simulink model "reducedorderobserver"  (R2023a)
settings: Solver=VariableStepAuto  StartTime=0.0  StopTime=10.0  RelTol=1e-3
values from neighbouring files (symbols this model uses):
  A = [0 0 1 0 0 ... (first row only)    [obsv_ctrb.m]    (also in reduced_order.m = [0 0 1 0)
  A_aa = A(1:2, 1:2)    [observer_design.m]
  A_ab = A(1:2, 3:4)    [observer_design.m]
  A_ba = A(3:4, 1:2)    [observer_design.m]
  A_bb = A(3:4, 3:4)    [observer_design.m]
  B = [0; 0; 0; 0; 1/L_a]    [obsv_ctrb.m]    (also in reduced_order.m = [0; 0; K_m/(J_m * R); 0])
  B_a = B(1:2, :)    [observer_design.m]
  B_b = B(3:4, :)    [observer_design.m]
  C = [0 1 0 0 0]    [obsv_ctrb.m]    (also in reduced_order.m = [0 1 0 0]; testobsv.m = [1 0 0 0 0])
  C_o = [1 0 0 0 ... (first row only)    [observer_design.m]
  K_cont_int = K_cont(1,1)    [polesplacement.m]
  K_cont_x = K_cont(1, 2:5)    [polesplacement.m]
  K_disc_int = K_disc(1,1)    [polesplacement.m]
  K_disc_x = K_disc(1, 2:5)    [polesplacement.m]
  L_r = place(A_bb', A_ab', [closest_pole, closest_pole+1])'    [observer_design.m]
  sys_disc = c2d(sys, min_sampling_time, "zoh")    [polesplacement.m]
  x1_bar = deg2rad(31.78)    [reduced_order.m]
  x2_bar = deg2rad(30)    [reduced_order.m]
undefined symbols (not defined in the file or in its folder): g, I_noload, init, K_m, l, m, min_sampling_time, R
libraries: simulink x2
settings Model: Creator=yunzh  LastModifiedBy=yunzh

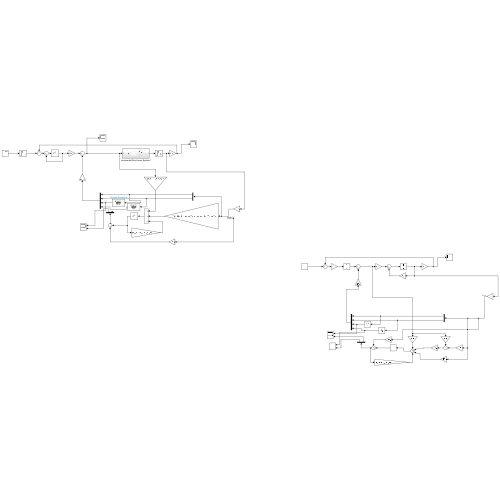
[thumbnail: Simulink's stored preview of the top-level diagram]
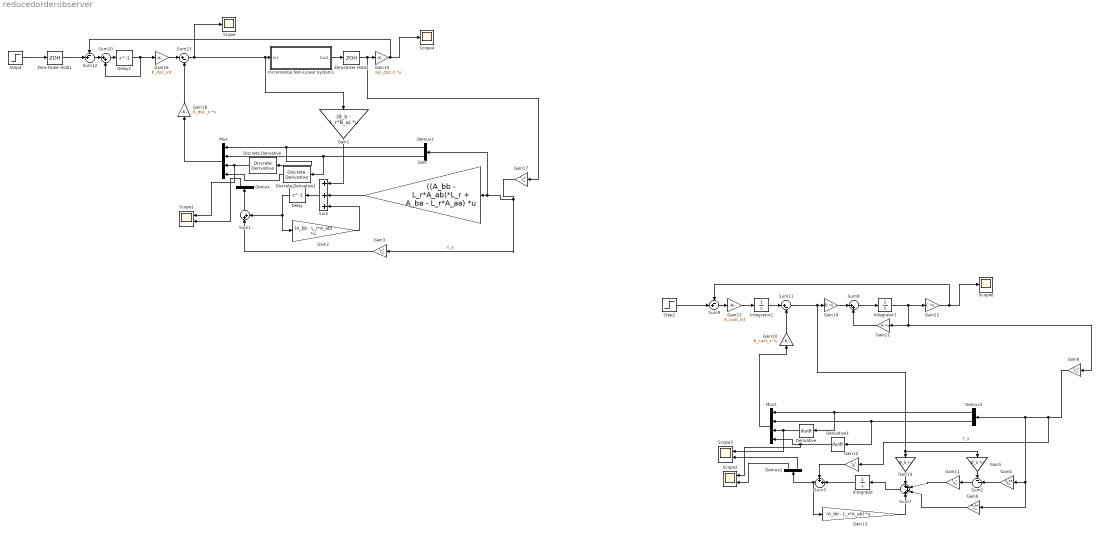
== system reducedorderobserver ==
  Delay : Delay  DelayLength=1
  Delay2 : Delay  DelayLength=1  SampleTime=min_sampling_time
  Demux{,1..3} (4 alike) : Demux  Outputs=2
  Derivative : Derivative
  Derivative1 : Derivative
  Discrete Derivative : simulink/Discrete/Discrete Derivative  gainval=1.0  ICPrevScaledInput=0.0  OutMin=[]  OutMax=[]  OutDataType=fixdt(1, 16)  OutScaling=2^-10  DoSatur=off
  Discrete Derivative1 : simulink/Discrete/Discrete Derivative  gainval=1.0  ICPrevScaledInput=0.0  OutMin=[]  OutMax=[]  OutDataType=fixdt(1, 16)  OutScaling=2^-10  DoSatur=off
  Gain : Gain  Gain=((A_bb - L_r*A_ab)*L_r + A_ba - L_r*A_aa)  Multiplication=Matrix(K*u)
  Gain1 : Gain  Gain=(B_b - L_r*B_a)  Multiplication=Matrix(K*u)
  Gain10 : Gain  Gain=B_b  Multiplication=Matrix(K*u)
  Gain11 : Gain  Gain=L_r  Multiplication=Matrix(K*u)
  Gain12 : Gain  Gain=L_r  Multiplication=Matrix(K*u)
  Gain13 : Gain  Gain=(A_bb - L_r*A_ab)  Multiplication=Matrix(K*u)
  Gain15 : Gain  Gain=sys_disc.C  Multiplication=Matrix(K*u)
  Gain16 : Gain  Gain=K_disc_int
  Gain17 : Gain  Gain=C_o  Multiplication=Matrix(K*u)
  Gain18 : Gain  Gain=K_disc_x  Multiplication=Matrix(K*u)
  Gain19 : Gain  Gain=B  Multiplication=Matrix(K*u)
  Gain2 : Gain  Gain=(A_bb - L_r*A_ab)  Multiplication=Matrix(K*u)
  Gain20 : Gain  Gain=K_cont_x  Multiplication=Matrix(K*u)
  Gain21 : Gain  Gain=A  Multiplication=Matrix(K*u)
  Gain22 : Gain  Gain=C  Multiplication=Matrix(K*u)
  Gain23 : Gain  Gain=K_cont_int
  Gain3 : Gain  Gain=L_r  Multiplication=Matrix(K*u)
  Gain4 : Gain  Gain=A_aa  Multiplication=Matrix(K*u)
  Gain5 : Gain  Gain=B_a  Multiplication=Matrix(K*u)
  Gain6 : Gain  Gain=A_ba  Multiplication=Matrix(K*u)
  Gain8 : Gain  Gain=C_o  Multiplication=Matrix(K*u)
  Incremental Non-Linear System1 : Subsystem
  Integrator : Integrator
  Integrator1 : Integrator
  Integrator2 : Integrator
  Mux : Mux
  Mux1 : Mux
  Scope : Scope
  Scope1 : Scope  NumInputPorts=2
  Scope2 : Scope  NumInputPorts=2
  Scope3 : Scope  NumInputPorts=2
  Scope4 : Scope
  Scope6 : Scope
  Step2 : Step  Time=0  After=0.5  SampleTime=0
  Step4 : Step  Time=0  After=deg2rad(15)  SampleTime=min_sampling_time
  Sum : Sum  Inputs=+++
  Sum1 : Sum  Inputs=|++
  Sum10 : Sum  Inputs=|++
  Sum11 : Sum  Inputs=|+-
  Sum12 : Sum  Inputs=-+|
  Sum13 : Sum  Inputs=|+-
  Sum2 : Sum  Inputs=--|
  Sum3 : Sum  Inputs=++|
  Sum7 : Sum  Inputs=++++
  Sum8 : Sum  Inputs=|++
  Sum9 : Sum  Inputs=-+|
  Zero-Order Hold1 : ZeroOrderHold  SampleTime=min_sampling_time
  Zero-Order Hold2 : ZeroOrderHold  SampleTime=-1
  wires:
  Gain18/1 -> Sum13/2
  Zero-Order Hold2/1 -> Gain17/1, Gain15/1
  Gain17/1 -> Gain3/1, Demux1/1, Gain/1  "X_a"
  Incremental Non-Linear System1/1(Out1) -> Zero-Order Hold2/1
  Sum13/1 -> Scope/1, Gain1/1, Incremental Non-Linear System1/1(In1)
  Zero-Order Hold1/1 -> Sum12/2
  Step4/1 -> Zero-Order Hold1/1
  Sum12/1 -> Sum10/1
  Gain15/1 -> Sum12/1, Scope4/1
  Gain16/1 -> Sum13/1
  Delay2/1 -> Sum10/2, Gain16/1
  Sum10/1 -> Delay2/1
  Gain1/1 -> Sum/1
  Gain/1 -> Sum/2
  Sum/1 -> Delay/1
  Delay/1 -> Gain2/1, Sum1/2
  Gain2/1 -> Sum/3
  Gain3/1 -> Sum1/1
  Sum1/1 -> Demux/1
  Mux/1 -> Gain18/1
  Demux1/1 -> Discrete Derivative/1, Mux/1
  Demux1/2 -> Discrete Derivative1/1, Mux/2
  Discrete Derivative/1 -> Scope1/1, Mux/3
  Discrete Derivative1/1 -> Mux/4
  Demux/1 -> Scope1/2
  Derivative1/1 -> Scope2/1, Mux1/4
  Derivative/1 -> Scope3/1, Mux1/3
  Demux3/1 -> Derivative/1, Mux1/1
  Demux3/2 -> Derivative1/1, Mux1/2
  Sum3/1 -> Gain13/1, Demux2/1
  Gain8/1 -> Gain12/1, Gain6/1, Gain4/1, Demux3/1  "X_a"
  Gain5/1 -> Sum2/1
  Gain4/1 -> Sum2/2
  Sum2/1 -> Gain11/1
  Gain10/1 -> Sum7/1
  Gain11/1 -> Sum7/2
  Integrator/1 -> Sum3/2
  Gain12/1 -> Sum3/1
  Sum7/1 -> Integrator/1
  Gain19/1 -> Sum8/1
  Gain20/1 -> Sum11/2
  Gain22/1 -> Sum9/1, Scope6/1
  Gain21/1 -> Sum8/2
  Step2/1 -> Sum9/2
  Sum8/1 -> Integrator1/1
  Integrator2/1 -> Sum11/1
  Integrator1/1 -> Gain8/1, Gain21/1, Gain22/1
  Sum9/1 -> Gain23/1
  Gain23/1 -> Integrator2/1
  Sum11/1 -> Gain5/1, Gain10/1, Gain19/1
  Mux1/1 -> Gain20/1
  Demux2/2 -> Scope3/2
  Demux2/1 -> Scope2/2
  Gain13/1 -> Sum7/4
  Gain6/1 -> Sum7/3

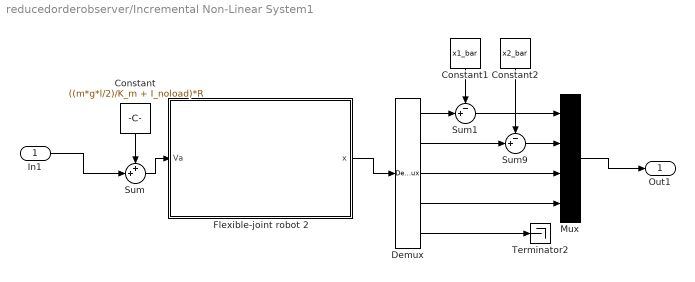
== system reducedorderobserver/Incremental Non-Linear System1 ==
  In1 : Inport
  Constant : Constant  Value=((m*g*l/2)/K_m + I_noload)*R
  Constant1 : Constant  Value=x1_bar
  Constant2 : Constant  Value=x2_bar
  Demux : Demux  Outputs=5
  Flexible-joint robot 2 : Subsystem
      mask Display: image('$imagefile'); % Use "Edit Image" on toolstrip to change.
  Mux : Mux
  Sum : Sum  Inputs=++|
  Sum1 : Sum  Inputs=-+|
  Sum9 : Sum  Inputs=-+|
  Terminator2 : Terminator
  Out1 : Outport
  wires:
  Flexible-joint robot 2/1(x) -> Demux/1
  Demux/1 -> Sum1/2
  Demux/2 -> Sum9/2
  Demux/5 -> Terminator2/1
  Sum/1 -> Flexible-joint robot 2/1(Va)
  Constant1/1 -> Sum1/1
  Sum9/1 -> Mux/2
  Constant2/1 -> Sum9/1
  Sum1/1 -> Mux/1
  Demux/4 -> Mux/4
  Demux/3 -> Mux/3
  Constant/1 -> Sum/1
  In1/1 -> Sum/2
  Mux/1 -> Out1/1

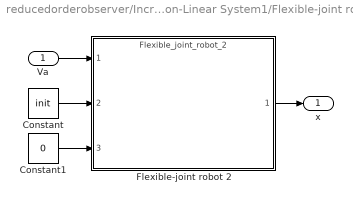
== system reducedorderobserver/Incremental Non-Linear System1/Flexible-joint robot 2 ==
  Va : Inport
  Constant : Constant  Value=init
  Constant1 : Constant  Value=0
  Flexible-joint robot 2 : ModelReference  ModelNameDialog=Flexible_joint_robot_2  ModelReferenceVersion=1.65  CopyOfModelProtected=on
  x : Outport
  wires:
  Va/1 -> Flexible-joint robot 2/1
  Constant1/1 -> Flexible-joint robot 2/3
  Constant/1 -> Flexible-joint robot 2/2
  Flexible-joint robot 2/1 -> x/1
